simulink model "clean"  (R2021b)
settings: Solver=VariableStepAuto  StartTime=0.0  StopTime=10.0  RelTol=1e-3
libraries: shared6dof x1
settings Model: Creator=josep  LastModifiedBy=josep

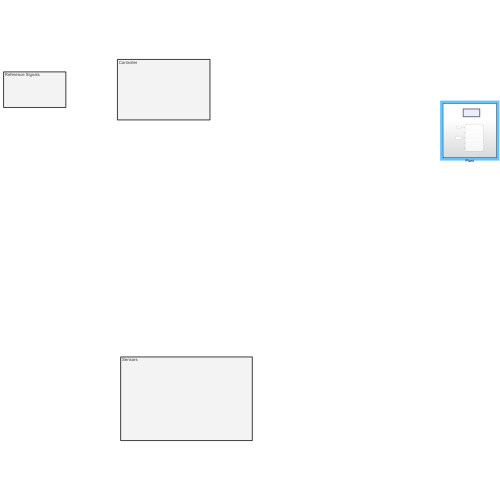
[thumbnail: Simulink's stored preview of the top-level diagram]
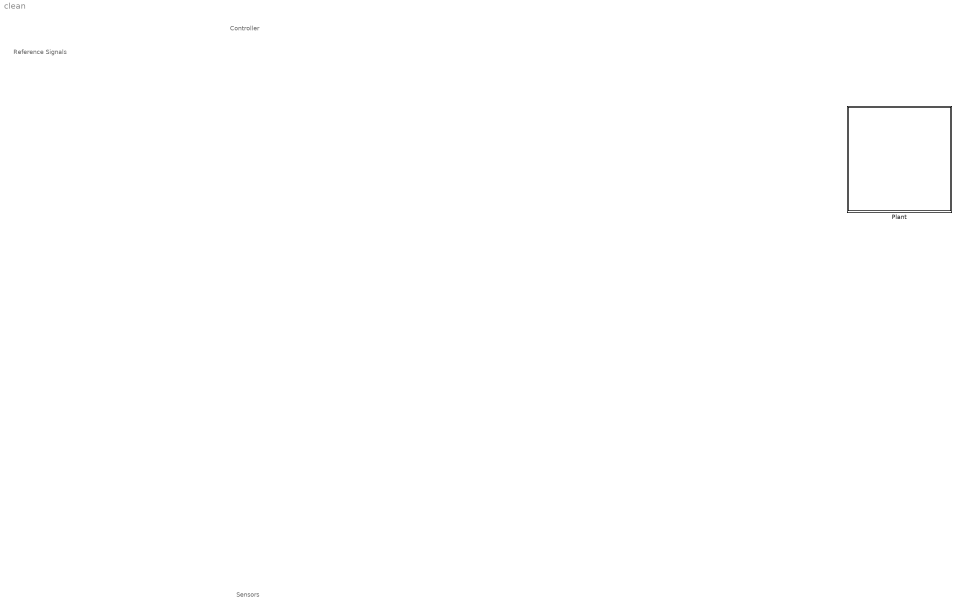
== system clean ==
  note: Sensors
  note: Reference Signals
  note: Controller
  Plant : Subsystem

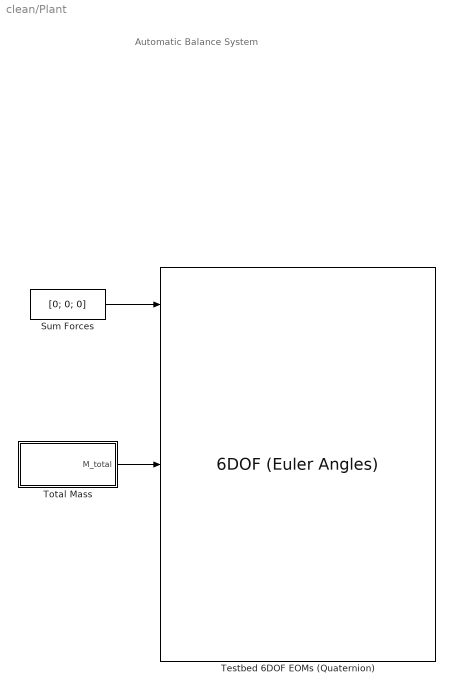
== system clean/Plant ==
  note: Automatic Balance System
  Sum Forces : Constant  Value=[0; 0; 0]  VectorParams1D=off
  Testbed 6DOF EOMs (Quaternion) : shared6dof/6DOF (Euler Angles)  units=Metric (MKS)  mtype=Custom Variable  rep=Quaternion  xme_0=[0 0 0]  Vm_0=[0 0 0]  eul_0=[0 0 0]  pm_0=[0 0 0]  mass_0=1.0  mass_e=0.5  mass_f=2.0  inertia=eye(3)  inertia_e=eye(3)  inertia_f=2*eye(3)  k_quat=1.0  vre_flag=off  abi_flag=off  aMode=0  xme_statename=''  Vm_statename=''  eul_statename=''  quat_statename=''  pm_statename=''  mass_statename=''
      settings: SourceProductBaseCode=AE,PW,DR,MT,UV,VE
  Total Mass : Subsystem
  wires:
  Sum Forces/1 -> Testbed 6DOF EOMs (Quaternion)/1
  Total Mass/1(M_total) -> Testbed 6DOF EOMs (Quaternion)/3

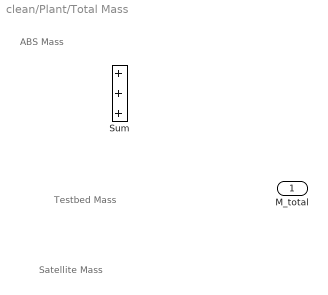
== system clean/Plant/Total Mass ==
  note: Satellite Mass
  note: Testbed Mass
  note: ABS Mass
  Sum : Sum  Inputs=+++
  M_total : Outport
